simulink model "attitudeError"  (R2023b)
settings: Solver=VariableStepAuto  StartTime=0.0  StopTime=Tfinal  RelTol=1e-3
libraries: matrix_library x1
settings Model: Creator=kristopherriordan  LastModifiedBy=kristopherriordan

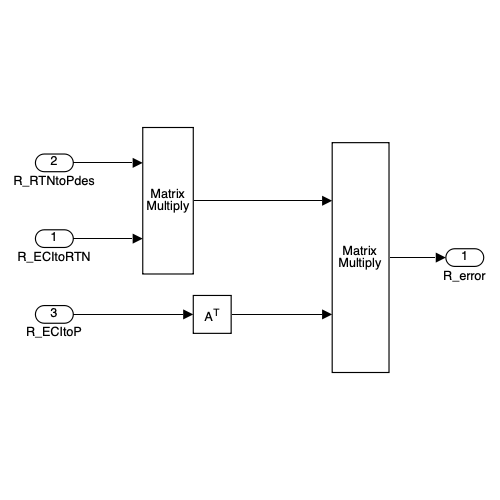
[thumbnail: Simulink's stored preview of the top-level diagram]
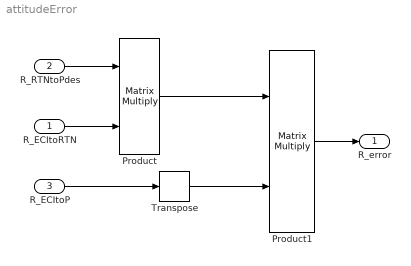
== system attitudeError ==
  R_ECItoRTN : Inport  PortDimensions=[3 3]
  R_RTNtoPdes : Inport  Port=2  PortDimensions=[3 3]
  R_ECItoP : Inport  Port=3  PortDimensions=[3 3]
  Product : Product  Multiplication=Matrix(*)
  Product1 : Product  Multiplication=Matrix(*)
  Transpose : matrix_library/Transpose
  R_error : Outport
  wires:
  R_ECItoRTN/1 -> Product/2
  R_RTNtoPdes/1 -> Product/1
  Product1/1 -> R_error/1
  R_ECItoP/1 -> Transpose/1
  Transpose/1 -> Product1/2
  Product/1 -> Product1/1
